simulink model "Semi_controlled_FW"  (R2021a)
settings: Solver=VariableStepAuto  StartTime=0.0  StopTime=0.5  RelTol=1e-3
libraries: spsThyristorLib x4, spsRMSLib x3, spsCurrentMeasurementLib x2, spsVoltageMeasurementLib x2, spsMeanLib x2, spsACVoltageSourceLib x1, spsDCVoltageSourceLib x1, spsSeriesRLCBranchLib x1, spspowerguiLib x1
settings Model: Creator=LEGION  LastModifiedBy=LEGION

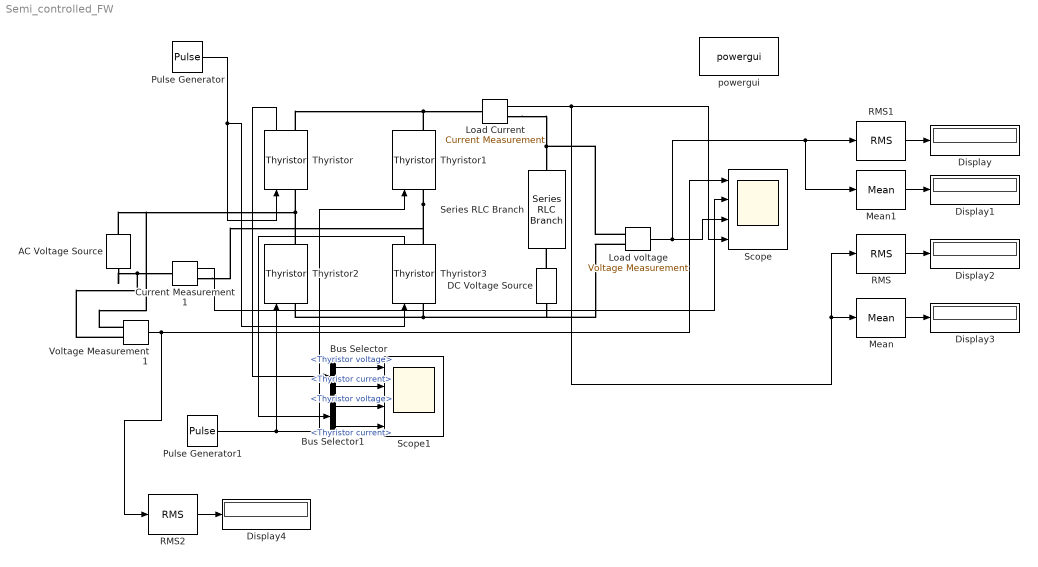
== system Semi_controlled_FW ==
  AC Voltage Source : spsACVoltageSourceLib/AC Voltage Source  Amplitude=230  Phase=0  Frequency=50  SampleTime=0  Measurements=None  BusType=swing  Pref=10e3  Qref=0  Qmin=-inf  Qmax=+inf
  Bus Selector : BusSelector  OutputSignals=Thyristor voltage,Thyristor current
  Bus Selector1 : BusSelector  OutputSignals=Thyristor voltage,Thyristor current
  Current Measurement1 : spsCurrentMeasurementLib/Current Measurement  PhasorSimulation=off  OutputType=Complex  PSBequivalent=0
  DC Voltage Source : spsDCVoltageSourceLib/DC Voltage Source  Amplitude=0  Measurements=None
  Display{,1..4} (5 alike) : Display
  "Load Current " : spsCurrentMeasurementLib/Current Measurement  PhasorSimulation=off  OutputType=Complex  PSBequivalent=0
  Load voltage : spsVoltageMeasurementLib/Voltage Measurement  PhasorSimulation=off  OutputType=Complex  PSBequivalent=0
  Mean : spsMeanLib/Mean  Freq=60  Vinit=0  Ts=0
  Mean1 : spsMeanLib/Mean  Freq=60  Vinit=0  Ts=0
  Pulse Generator : DiscretePulseGenerator  PulseType=Time based  Period=0.01  PulseWidth=5  PhaseDelay=45*(0.01/180)
  Pulse Generator1 : DiscretePulseGenerator  PulseType=Time based  Period=0.01  PulseWidth=5  PhaseDelay=(180+45)*(0.01/180)
  RMS : spsRMSLib/RMS  TrueRMS=on  Freq=60  RMSInit=120  Ts=0
  RMS1 : spsRMSLib/RMS  TrueRMS=on  Freq=60  RMSInit=120  Ts=0
  RMS2 : spsRMSLib/RMS  TrueRMS=on  Freq=60  RMSInit=120  Ts=0
  Scope : Scope  NumInputPorts=4
  Scope1 : Scope  NumInputPorts=4
  Series RLC Branch : spsSeriesRLCBranchLib/Series RLC Branch  LConnTagsString=__new0  RConnTagsString=__new0  BranchType=RL  Resistance=12.5  Inductance=1  SetiL0=off  InitialCurrent=0  Capacitance=1e-6  Setx0=off  InitialVoltage=0  Measurements=None
  Thyristor{,1..3} (4 alike) : spsThyristorLib/Thyristor  Ron=0.001  Lon=0  Vf=1.5  IC=0  Rs=500  Cs=250e-9  Measurements=on
  Voltage Measurement1 : spsVoltageMeasurementLib/Voltage Measurement  PhasorSimulation=off  OutputType=Complex  PSBequivalent=0
  powergui : spspowerguiLib/powergui  Priority=1  SimulationMode=Continuous  SampleTime=50e-6  frequency=60  Iterations=50  frequencyindice=50  Pbase=100e6  ErrMax=1e-4  UnitsV=kV  UnitsW=MW  buscounter=0  FunctionMessages=off  echomessages=off  EnableUseOfTLC=off  CurrentSourceSwitches=off  DisableSnubberDevices=off  DisableRonSwitches=off  DisableVfSwitches=off  DisplayEquations=off  AutomaticDiscreteSolvers=off  SolverType=Tustin/Backward Euler (TBE)  Interpol=off  ExternalGateDelay=off  methode=off  Ts=100  x0status=blocks  SPID=on  SwTol=0  HookPort=off  NonlinearTolerance=1e-4  nMaxIteration=100  ContinueOnMaxIteration=off  RestoreLinks=warning  ResistiveCurrentMeasurement=off  Frange=[0:2:500]  Ylog=off  Xlog=on  ShowGrid=off  save=off  variable=ZData  structure=0  ZoomFFT=off  StartTime=0.0  cycles=1  DisplayStyle=1  fundamental=60  FreqAxis=off  MaxFrequency=1000  frequencyindicesteady=1  RmsSteady=1  display=off
  wires:
  Voltage Measurement1/1 -> RMS2/1, Scope/1
  Current Measurement1/1 -> Scope/2
  Load voltage/1 -> Mean1/1, RMS1/1, Scope/3
  "Load Current "/1 -> Mean/1, RMS/1, Scope/4
  Bus Selector1/1 -> Scope1/3  "<Thyristor voltage>"
  Bus Selector1/2 -> Scope1/4  "<Thyristor current>"
  Bus Selector/1 -> Scope1/1  "<Thyristor voltage>"
  Bus Selector/2 -> Scope1/2  "<Thyristor current>"
  Thyristor/1 -> Bus Selector/1
  Thyristor3/1 -> Bus Selector1/1
  Pulse Generator/1 -> Thyristor3/1, Thyristor/1
  Pulse Generator1/1 -> Thyristor1/1, Thyristor2/1
  Mean/1 -> Display3/1
  RMS/1 -> Display2/1
  RMS1/1 -> Display/1
  Mean1/1 -> Display1/1
  RMS2/1 -> Display4/1
  connections:
  Voltage Measurement1/LConn1 -- AC Voltage Source/RConn1 -- Thyristor2/RConn1 -- Thyristor/LConn1
  Thyristor1/LConn1 -- Thyristor3/RConn1 -- Current Measurement1/RConn1
  Load voltage/LConn2 -- DC Voltage Source/LConn1 -- Thyristor3/LConn1 -- Thyristor2/LConn1
  Thyristor1/RConn1 -- "Load Current "/LConn1 -- Thyristor/RConn1
  "Load Current "/RConn1 -- Load voltage/LConn1 -- Series RLC Branch/LConn1
  DC Voltage Source/RConn1 -- Series RLC Branch/RConn1
  AC Voltage Source/LConn1 -- Voltage Measurement1/LConn2 -- Current Measurement1/LConn1
